simulink model "sft_ut"  (Simulink 8.1)
settings: Solver=FixedStepDiscrete  StartTime=0.0  StopTime=10  FixedStep=5e-3  RelTol=1e-3
PostLoadFcn:
  | , if any(exist('dsrtsu_mdlpostloadfcn', 'file') == [2, 3, 6]), try dsrtsu_mdlpostloadfcn('Execute', bdroot); catch fprintf('Error in PostLoadFcn (dsrtsu_mdlpostloadfcn) for model "%s":\n %s\n', bdroot, lasterr); end, end,
libraries: siltestlib x23, sft x1
settings Model: DSRTSU_INTERNAL_RTI_VER=450  DSRTSU_INTERNAL_RTI_TYPE=rti1401  RTICANMMDATA=struct('GeneralSetupData',struct('modelroot','D:\ELN150201_TAIWAN\trunk\AdasDragon\software\sw_development\arch\app\ifo','generalsettings',struct('filesettings',struct('destfolder',struct('Name','RTICANMM_FILES','Check',1),'buildfolder',struct('Name','.','Check',1),'AbsDestfolder',struct('Name','D:\ELN150201_TAIWAN\trunk\AdasDragon\software\sw_development\arch\app\ifo\RTICANMM_FILES'),'AbsBuildfolder',struct('Name','D:\ELN150201_TAIWAN\trunk\AdasDragon\software\sw_development\arch\app\ifo'))),'options',struct('addpaths',1,'rmpaths',1,'addtrcexclusion',logical(1),'cannavigator',struct('checkmonitoring',0),'show_usrtrc',0,'use_usrtrc',0),'advanced',struct('options',[1 1 1 1 1 1 1 1 1 1 1 1 1 1 1 1 1 1 1 1 1 1 1 1 1 1 1 1 1 1 1 1 1 1 1 1 1 1 1 1 1 1 1 1 1 1 1 1 1 1 1 1 1 1 1 1 1 1 1 1 1 1 1 1 1 1 1 1 1 1 1 1 1 1 1 1 1 1 1 1 1 1 1 1 1 1 1 1 1 1 1 1 1 1 1 1 1 1 1 1]),'MPSetup',{{}},'modelname','sft_ut','block','sft_ut'))  DSRTSU_INTERNAL_RTIFPGA=40  Creator=tescamilla  LastModifiedBy=AT015555  BufferReuse=off
settings DataIOCC: SignalLoggingSaveFormat=Dataset
settings OptimizationCC: BlockReduction=off  OptimizeBlockIOStorage=off  BufferReuse=off  ExpressionFolding=off  ExpressionDepthLimit=128  LocalBlockOutputs=off
settings DebuggingCC: FcnCallInpInsideContextMsg=EnableAllAsError
settings HardwareCC: ProdIntDivRoundTo=Zero  ProdEndianess=BigEndian  ProdHWDeviceType=Generic->Custom  TargetIntDivRoundTo=Zero  TargetEndianess=BigEndian  TargetHWDeviceType=Generic->Custom
settings RTWCC: SystemTargetFile=rti1401.tlc  MakeCommand=make_rti  TemplateMakefile=rti1401.tmf  Description=dSPACE DS1401 Hardware Platform  ProcessScript=rti1401_make_rtw_hook
settings STFCustomTargetCC: CodeReplacementLibrary=ANSI_C  ParMdlRefBuildCompliant=on  GeneratePreprocessorConditionals=Disable all  MatFileLogging=on  SystemTargetFile=rti1401.tlc
settings GRTTargetCC: CompOptLevelCompliant=off  ConcurrentExecutionCompliant=off  ExtModeMexFile=noextcomm
settings CustomProperty: DataType=RTWOptions_EnumType_C__Program Files (x86)_dSPACE RCPHIL 2014-B_MATLAB_RTI_RTI1401_TLC_rti1401_1InitialSimState  Value=RUN
settings EnumStrPairs: String=RUN

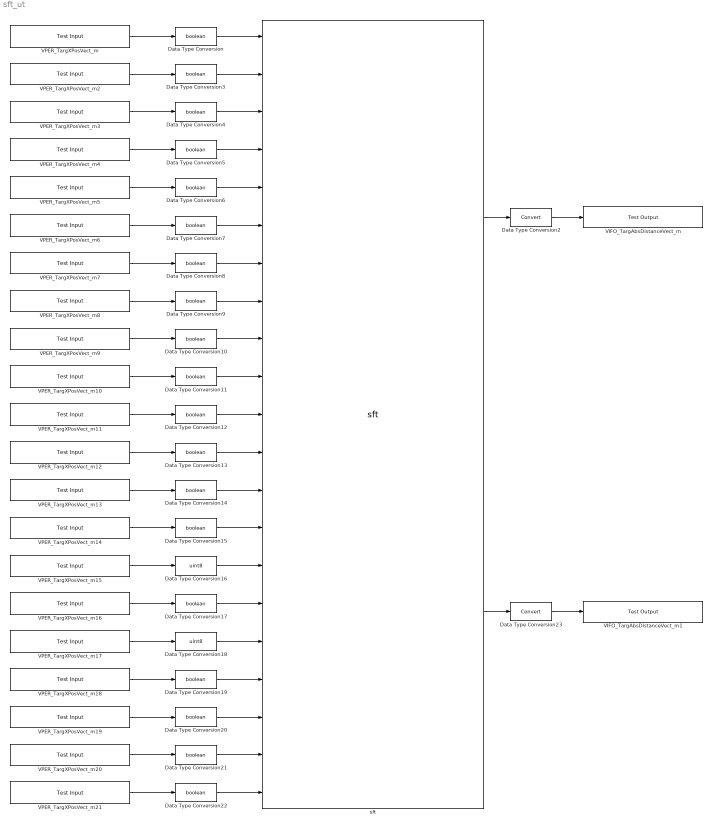
== system sft_ut ==
  Data Type Conversion{,3..15,17,19..22} (19 alike) : DataTypeConversion  OutDataTypeStr=boolean
  Data Type Conversion16 : DataTypeConversion  OutDataTypeStr=uint8
  Data Type Conversion18 : DataTypeConversion  OutDataTypeStr=uint8
  Data Type Conversion2 : DataTypeConversion
  Data Type Conversion23 : DataTypeConversion
  VIFO_TargAbsDistanceVect_m : siltestlib/Test Output  varname=VIFO_DriverSafetyStatusOk_flg  sampletime=-1
  VIFO_TargAbsDistanceVect_m1 : siltestlib/Test Output  varname=VIFO_VehicleStatusOk_flg  sampletime=-1
  VPER_TargXPosVect_m : siltestlib/Test Input  varname=VDINR_SeatBeltNOTFasten_flg  sampletime=0.005
  VPER_TargXPosVect_m10 : siltestlib/Test Input  varname=VDINR_HWAccelPedalPosnValid_flg  sampletime=0.005
  VPER_TargXPosVect_m11 : siltestlib/Test Input  varname=VDINR_DriverBrakPedalOnValid_flg  sampletime=0.005
  VPER_TargXPosVect_m12 : siltestlib/Test Input  varname=VDINR_NowGearPosnValid_flg  sampletime=0.005
  VPER_TargXPosVect_m13 : siltestlib/Test Input  varname=VDINR_ESCFault_flg  sampletime=0.005
  VPER_TargXPosVect_m14 : siltestlib/Test Input  varname=VDINR_ABSFault_flg  sampletime=0.005
  VPER_TargXPosVect_m15 : siltestlib/Test Input  varname=VDINR_EMSOpState_enum  sampletime=0.005
  VPER_TargXPosVect_m16 : siltestlib/Test Input  varname=VDINR_EPASMlLReq_flg  sampletime=0.005
  VPER_TargXPosVect_m17 : siltestlib/Test Input  varname=VDINR_TCMFaultStatus_enum  sampletime=0.005
  VPER_TargXPosVect_m18 : siltestlib/Test Input  varname=VDINR_DriverDoorOpen_flg  sampletime=0.005
  VPER_TargXPosVect_m19 : siltestlib/Test Input  varname=VDINR_PassengerDoorOpen_flg  sampletime=0.005
  VPER_TargXPosVect_m2 : siltestlib/Test Input  varname=VDINR_VehCrashed_flg  sampletime=0.005
  VPER_TargXPosVect_m20 : siltestlib/Test Input  varname=VDINR_LRDoorOpen_flg  sampletime=0.005
  VPER_TargXPosVect_m21 : siltestlib/Test Input  varname=VDINR_RRDoorOpen_flg  sampletime=0.005
  VPER_TargXPosVect_m3 : siltestlib/Test Input  varname=VDINR_TCSActive_flg  sampletime=0.005
  VPER_TargXPosVect_m4 : siltestlib/Test Input  varname=VDINR_VehSpdValid_flg  sampletime=0.005
  VPER_TargXPosVect_m5 : siltestlib/Test Input  varname=VDINR_LongAccelValid_flg  sampletime=0.005
  VPER_TargXPosVect_m6 : siltestlib/Test Input  varname=VDINR_LatAccelValid_flg  sampletime=0.005
  VPER_TargXPosVect_m7 : siltestlib/Test Input  varname=VDINR_YawRateValid_flg  sampletime=0.005
  VPER_TargXPosVect_m8 : siltestlib/Test Input  varname=VDINR_SteerAngleValid_flg  sampletime=0.005
  VPER_TargXPosVect_m9 : siltestlib/Test Input  varname=VDINR_SteerSpeedValid_flg  sampletime=0.005
  sft : sft/sft
  wires:
  Data Type Conversion2/1 -> VIFO_TargAbsDistanceVect_m/1
  VPER_TargXPosVect_m/1 -> Data Type Conversion/1
  Data Type Conversion/1 -> sft/1
  sft/1 -> Data Type Conversion2/1
  VPER_TargXPosVect_m2/1 -> Data Type Conversion3/1
  Data Type Conversion3/1 -> sft/2
  VPER_TargXPosVect_m3/1 -> Data Type Conversion4/1
  Data Type Conversion4/1 -> sft/3
  VPER_TargXPosVect_m4/1 -> Data Type Conversion5/1
  Data Type Conversion5/1 -> sft/4
  VPER_TargXPosVect_m5/1 -> Data Type Conversion6/1
  Data Type Conversion6/1 -> sft/5
  VPER_TargXPosVect_m6/1 -> Data Type Conversion7/1
  Data Type Conversion7/1 -> sft/6
  VPER_TargXPosVect_m7/1 -> Data Type Conversion8/1
  VPER_TargXPosVect_m8/1 -> Data Type Conversion9/1
  VPER_TargXPosVect_m9/1 -> Data Type Conversion10/1
  VPER_TargXPosVect_m10/1 -> Data Type Conversion11/1
  VPER_TargXPosVect_m11/1 -> Data Type Conversion12/1
  VPER_TargXPosVect_m12/1 -> Data Type Conversion13/1
  VPER_TargXPosVect_m13/1 -> Data Type Conversion14/1
  VPER_TargXPosVect_m14/1 -> Data Type Conversion15/1
  VPER_TargXPosVect_m15/1 -> Data Type Conversion16/1
  VPER_TargXPosVect_m16/1 -> Data Type Conversion17/1
  VPER_TargXPosVect_m17/1 -> Data Type Conversion18/1
  VPER_TargXPosVect_m18/1 -> Data Type Conversion19/1
  VPER_TargXPosVect_m19/1 -> Data Type Conversion20/1
  VPER_TargXPosVect_m20/1 -> Data Type Conversion21/1
  VPER_TargXPosVect_m21/1 -> Data Type Conversion22/1
  Data Type Conversion22/1 -> sft/21
  Data Type Conversion12/1 -> sft/11
  Data Type Conversion11/1 -> sft/10
  Data Type Conversion10/1 -> sft/9
  Data Type Conversion9/1 -> sft/8
  Data Type Conversion20/1 -> sft/19
  Data Type Conversion14/1 -> sft/13
  Data Type Conversion13/1 -> sft/12
  Data Type Conversion15/1 -> sft/14
  Data Type Conversion17/1 -> sft/16
  Data Type Conversion16/1 -> sft/15
  Data Type Conversion8/1 -> sft/7
  Data Type Conversion19/1 -> sft/18
  Data Type Conversion18/1 -> sft/17
  Data Type Conversion21/1 -> sft/20
  Data Type Conversion23/1 -> VIFO_TargAbsDistanceVect_m1/1
  sft/2 -> Data Type Conversion23/1
